simulink model "lab"  (R2024a)
settings: Solver=ode4  StartTime=0.0  StopTime=50  FixedStep=0.001  RelTol=1e-3
undefined symbols (not defined in the file or in its folder): sigbuilder_block
libraries: slpidlib x1
settings Model: Creator=colom  LastModifiedBy=guilherme
settings SolverCC: AlgebraicLoopSolver=TrustRegion  AutoInsertRateTranBlk=on
settings OptimizationCC: LifeSpan=inf
settings DebuggingCC: SFExecutionAtInitializationDiag=none  ArithmeticOperatorsInVariantConditions=warning
settings HardwareCC: ProdBitPerSizeT=32  ProdBitPerPtrDiffT=32  ProdWordSize=32  ProdHWDeviceType=Specified
settings SFSimCC: CustomCodeUndefinedFunction=UseInterfaceOnly
settings RTWCC: GPUComputeCapability=3.5
settings CodeAppCC: StateflowObjectComments=on

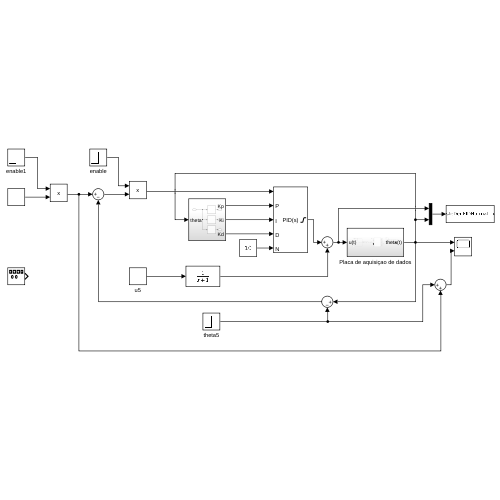
[thumbnail: Simulink's stored preview of the top-level diagram]
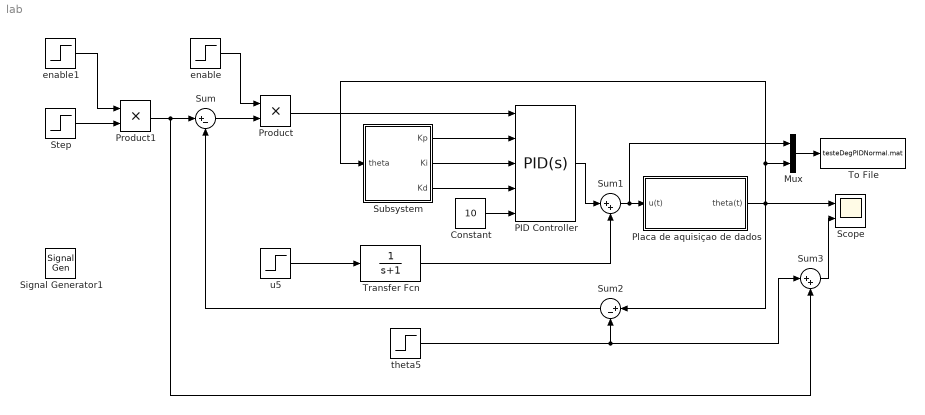
== system lab ==
  Constant : Constant  Value=10
  Mux : Mux  Inputs=2
  PID Controller : slpidlib/PID Controller  Controller=PID  Form=Parallel  TimeDomain=Continuous-time  UseExternalTs=off  SampleTime=-1  IntegratorMethod=Forward Euler  FilterMethod=Forward Euler  ControllerParametersSource=external  P=-0.9  I=60  UseKiTs=off  D=2.15  UseExternalDerivativeSource=off  N=10  UseFilter=on  TunerSelectOption=Transfer Function Based (PID Tuner App)  InitialConditionSource=internal  InitialConditionForIntegrator=0  InitialConditionForFilter=0  DifferentiatorICPrevScaledInput=0  ExternalReset=none  TrackingMode=off  Kt=1  LimitOutput=on  SatLimitsSource=internal  UpperSaturationLimit=85  LowerSaturationLimit=-15  LinearizeAsGain=on  AntiWindupMode=back-calculation  Kb=1  LimitIntegrator=off  UpperIntegratorSaturationLimit=inf  LowerIntegratorSaturationLimit=-inf  POutMin=[]  POutMax=[]  IOutMin=[]  IOutMax=[]  DOutMin=[]  DOutMax=[]  NOutMin=[]  NOutMax=[]  SumOutMin=[]  SumOutMax=[]  SaturationOutMin=[]  SaturationOutMax=[]  PParamMin=[]  PParamMax=[]  IParamMin=[]  IParamMax=[]  DParamMin=[]  DParamMax=[]  NParamMin=[]  NParamMax=[]  KbParamMin=[]  KbParamMax=[]  KtParamMin=[]  KtParamMax=[]  KbOutMin=[]  KbOutMax=[]  KtOutMin=[]  KtOutMax=[]  IntegratorOutMin=[]  IntegratorOutMax=[]  FilterOutMin=[]  FilterOutMax=[]  SumI1OutMin=[]  SumI1OutMax=[]  SumI2OutMin=[]  SumI2OutMax=[]  SumI3OutMin=[]  SumI3OutMax=[]  SumI4OutMin=[]  SumI4OutMax=[]  SumDOutMin=[]  SumDOutMax=[]  DifferentiatorOutMin=[]  DifferentiatorOutMax=[]  FilterDiffOutCoefMin=[]  FilterDiffOutCoefMax=[]  ReciprocalOutMin=[]  ReciprocalOutMax=[]  SumDenOutMin=[]  SumDenOutMax=[]  SumNumOutMin=[]  SumNumOutMax=[]  DivideOutMin=[]  DivideOutMax=[]  UdiffTsProdOutMin=[]  UdiffTsProdOutMax=[]  NTsProdOutMin=[]  NTsProdOutMax=[]  UintegralTsProdOutMin=[]  UintegralTsProdOutMax=[]  UngainTsProdOutMin=[]  UngainTsProdOutMax=[]  ClampingZeroOutDataTypeStr=Inherit: Inherit via back propagation  ClampingZeroOutMin=[]  ClampingZeroOutMax=[]  FilterDenConstantOutDataTypeStr=Inherit: Inherit via back propagation  FilterDenConstantOutMin=[]  FilterDenConstantOutMax=[]  PCopyOutDataTypeStr=Inherit: Inherit via back propagation  PCopyOutMin=[]  PCopyOutMax=[]  NCopyOutDataTypeStr=Inherit: Inherit via back propagation  NCopyOutMin=[]  NCopyOutMax=[]  IntegratorContinuousStateAttributes=''  IntegratorStateMustResolveToSignalObject=off  IntegratorRTWStateStorageClass=Auto  FilterContinuousStateAttributes=''  FilterStateMustResolveToSignalObject=off  FilterRTWStateStorageClass=Auto  ParallelPVariant=ExternalParameters  IdealPVariant=Disabled  IVariant=ExternalParameters  DVariant=ExternalParameters  IntegratorVariant=Continuous  SatVariant=Enabled  AWVariant=BackCalculation  PCopyVariant=Disabled  TRVariant=Disabled  FdbkBlocksVariant=Forward  IdealPFdbkVariant=Disabled  SatFdbkVariant=Disabled  DerivativeFilterVariant=ContFilter  NVariant=ExternalParameters  NCopyVariant=Disabled  FilterICVariant=InternalICsFilter  IntegratorICVariant=InternalICs  ExternalResetVariant=Disabled  TRSumVariant=Passthrough  SumFdbkVariant=Disabled  SumVariant=Sum_PID  TsampFilterVariant=InternalTs  TsampNgainVariant=Passthrough  TsampIntegralVariant=Disabled_SignalSpec  ExternalSaturationOutDataTypeStr=Inherit: Same as second input  DerivativeSourceVariant=ErrorSignal
  Placa de aquisiçao de dados : Subsystem
  Product : Product
  Product1 : Product
  Scope : Scope  NumInputPorts=2
  Signal Generator1 : SignalGenerator  WaveForm=square  Amplitude=deg2rad(10)  Frequency=0.4  Units=rad/sec
  Step : Step  Time=23  After=deg2rad(42)  SampleTime=0
  Subsystem : Subsystem
  Sum : Sum  Inputs=|+-
  Sum1 : Sum  Inputs=|++
  Sum2 : Sum  Inputs=|+-
  Sum3 : Sum  Inputs=|++
  To File : ToFile  Filename=testeDegPIDNormal.mat
      settings: Decimation=3
  Transfer Fcn : TransferFcn  Denominator=[1 1]
  enable : Step  Time=23  SampleTime=0
  enable1 : Step  Time=0  SampleTime=0
  theta5 : Step  Time=16  After=0  SampleTime=0
  u5 : Step  Time=16  After=0  SampleTime=0
  wires:
  Placa de aquisiçao de dados/1(theta(t)) -> Scope/1, Sum2/1, Subsystem/1(theta), Mux/2
  Mux/1 -> To File/1
  u5/1 -> Transfer Fcn/1
  Sum2/1 -> Sum/2
  theta5/1 -> Sum3/1, Sum2/2
  Product/1 -> PID Controller/1
  enable/1 -> Product/1
  Transfer Fcn/1 -> Sum1/2
  Sum1/1 -> Mux/1, Placa de aquisiçao de dados/1(u(t))
  Sum3/1 -> Scope/2
  Sum/1 -> Product/2
  PID Controller/1 -> Sum1/1
  Subsystem/1(Kp) -> PID Controller/2
  Subsystem/2(Ki) -> PID Controller/3
  Subsystem/3(Kd) -> PID Controller/4
  Constant/1 -> PID Controller/5
  Step/1 -> Product1/2
  enable1/1 -> Product1/1
  Product1/1 -> Sum3/2, Sum/1

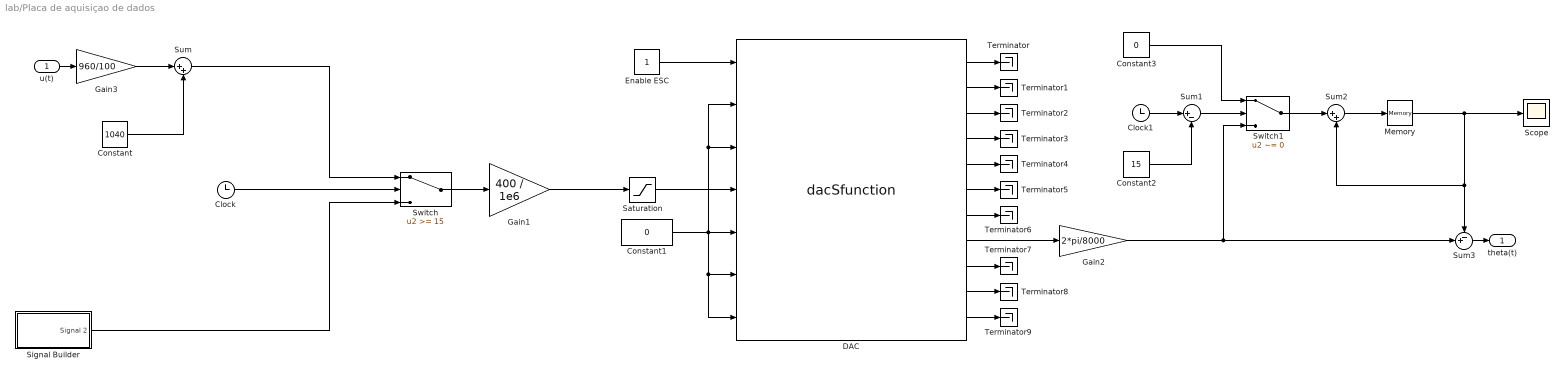
== system lab/Placa de aquisiçao de dados ==
  u(t) : Inport
  Clock : Clock
  Clock1 : Clock
  Constant : Constant  Value=1040
  Constant1 : Constant  Value=0
  Constant2 : Constant  Value=15
  Constant3 : Constant  Value=0
  DAC : S-Function  FunctionName=dacSfunction  Parameters=serialPort,sampleTime,gpioOutCh1FinalState,gpioOutCh2FinalState,gpioOutCh3FinalState,pwmFrequency,pwmCh1FinalDuty,pwmCh2FinalDuty,pwmCh3FinalDuty,pwmCh4FinalDuty,enc1Mode,enc1ResetCount,enc1Direction,enc1Quadrature,enc1Filter,enc2Mode,enc2ResetCount,enc2Direction,enc2Quadrature,enc2Filter,enc3Mode,enc3ResetCount,enc3Direction,enc3Quadrature,enc3Filter  SFunctionDeploymentMode=off  EnableBusSupport=off  mask{serialPort='/dev/ttyACM0', sampleTime=5, gpioOutCh1FinalState=Low, gpioOutCh2FinalState=Low, gpioOutCh3FinalState=Low, pwmFrequency=400, pwmCh1FinalDuty=0, pwmCh2FinalDuty=0, pwmCh3FinalDuty=0, pwmCh4FinalDuty=0, enc1Mode=Counter, enc1Direction=Counter Clock Wise is positive, enc1Quadrature=High resolution, enc1Filter=15, enc1ResetCount=on, enc2Mode=Counter, enc2Direction=Counter Clock Wise is positive, enc2Quadrature=High resolution, enc2Filter=15, enc2ResetCount=off, enc3Mode=Counter, enc3Direction=Clock Wise is positive, enc3Quadrature=High resolution, enc3Filter=15, enc3ResetCount=off}
      mask prompts: serialPort "Serial port"; sampleTime "Sample time (ms)"; gpioOutCh1FinalState "Final state"; gpioOutCh2FinalState "Final state"; gpioOutCh3FinalState "Final state"; pwmFrequency "Frequency (Hz)"; pwmCh1FinalDuty "Final duty"; pwmCh2FinalDuty "Final duty"; pwmCh3FinalDuty "Final duty"; pwmCh4FinalDuty "Final duty"; enc1Mode "Mode"; enc1Direction "Direction"; enc1Quadrature "Resolution"; enc1Filter "Filter"; enc1ResetCount "Reset count"; enc2Mode "Mode"; enc2Direction "Direction"; enc2Quadrature "Resolution"; enc2Filter "Filter"; enc2ResetCount "Reset count"; enc3Mode "Mode"; enc3Direction "Direction"; enc3Quadrature "Resolution"; enc3Filter "Filter"; enc3ResetCount "Reset count"
      mask init:
      | % The first list item is initiated with 1 and not 0
      mask TypeOptions gpioOutCh1FinalState: Low | High
      mask TypeOptions gpioOutCh2FinalState: Low | High
      mask TypeOptions gpioOutCh3FinalState: Low | High
      mask TypeOptions enc1Mode: Counter | Time measurement
      mask TypeOptions enc1Direction: Counter Clock Wise is positive | Clock Wise is positive
      mask TypeOptions enc1Quadrature: Low resolution | High resolution
      mask TypeOptions enc2Mode: Counter | Time measurement
      mask TypeOptions enc2Direction: Counter Clock Wise is positive | Clock Wise is positive
      mask TypeOptions enc2Quadrature: Low resolution | High resolution
      mask TypeOptions enc3Mode: Counter | Time measurement
      mask TypeOptions enc3Direction: Counter Clock Wise is positive | Clock Wise is positive
      mask TypeOptions enc3Quadrature: Low resolution | High resolution
      mask DialogControl DescTextVar Prompt: %<MaskDescription> OpenDAC configuration
      mask DialogControl Container18 Prompt: General configuration
      mask DialogControl Container8 Prompt: GPIO Output
      mask DialogControl Container19 Prompt: Channel 1
      mask DialogControl Container22 Prompt: Channel 2
      mask DialogControl Container21 Prompt: Channel 3
      mask DialogControl Container6 Prompt: PWM
      mask DialogControl Container42 Prompt: General
      mask DialogControl Container43 Prompt: Channel 1
      mask DialogControl pwmCh1FinalDuty Tooltip: 0 - 100%
      mask DialogControl Container11 Prompt: Channel 2
      mask DialogControl pwmCh2FinalDuty Tooltip: 0 - 100%
      mask DialogControl Container12 Prompt: Channel 3
      mask DialogControl pwmCh3FinalDuty Tooltip: 0 - 100%
      mask DialogControl Container13 Prompt: Channel 4
      mask DialogControl pwmCh4FinalDuty Tooltip: 0 - 100%
      mask DialogControl Container4 Prompt: Encoders
      mask DialogControl Container35 Prompt: Encoder 1
      mask DialogControl enc1Quadrature Tooltip: In pulse count mode, Low resolution implements X2 quadrature and High resolution implements X4 quadrature. In time measurement mode, Low Resolution measure time between two rise edges on CHA and High Resolution measure time between rise and fall edges on CHA.
      mask DialogControl Container36_copy Prompt: Encoder 2
      mask DialogControl enc2Quadrature Tooltip: In pulse count mode, Low resolution implements X2 quadrature and High resolution implements X4 quadrature. In time measurement mode, Low Resolution measure time between two rise edges on CHA and High Resolution measure time between rise and fall edges on CHA.
      mask DialogControl Container36 Prompt: Encoder 3
      mask DialogControl enc3Quadrature Tooltip: In pulse count mode, Low resolution implements X2 quadrature and High resolution implements X4 quadrature. In time measurement mode, Low Resolution measure time between two rise edges on CHA and High Resolution measure time between rise and fall edges on CHA.
      mask Display:
      | % Give names to the input ports
      | port_label('input', 1, 'Digital Out CH1 (PC15)');
      | port_label('input', 2, 'Digital Out CH2 (PC14)');
      | port_label('input', 3, 'Digital Out CH3 (PC13)');
      | port_label('input', 4, 'PWM CH1 (PB6)');
      | port_label('input', 5, 'PWM CH2 (PB7)');
      | port_label('input', 6, 'PWM CH3 (PB8)');
      | port_label('input', 7, 'PWM CH4 (PB9)');
      | 
      | % Give names to the output ports
      | port_label('output', 1, 'Digital In CH1 (PB12)');
      | port_label('output', 2, 'Digital In CH2 (PB13)');
      | port_label('output', 3, 'Digital In CH3 (PB14)');
      | port_label('output', 4, 'Analog In CH1 (PA0)');
      | port_label('output', 5, 'Analog In CH2 (PA1)');
      | port_label('output', 6, 'Analog In CH3 (PA4)');
      | port_label('output', 7, 'Analog In CH4 (PB0)');
      | port_label('output', 8, 'Encoder 1 (PA8/PA9)');
      | port_label('output', 9, 'Encoder 2 (PA15/PB3)');
      | port_label('output', 10, 'Encoder 3 (PB4/PB5)');
      | port_label('output', 11, 'Real Time Clock');
  Enable ESC : Constant
  Gain1 : Gain  Gain=400 / 1e6
  Gain2 : Gain  Gain=2*pi/8000
  Gain3 : Gain  Gain=960/100
  Memory : Memory
  Saturation : Saturate  UpperLimit=0.8  LowerLimit=0
  Scope : Scope
  Signal Builder : Subsystem  Tag=STV Subsys  LoadFcn=sigbuilder_block('load');  StartFcn=sigbuilder_block('start');  StopFcn=sigbuilder_block('stop');  ClipboardFcn=sigbuilder_block('clipboard');  mask(Sigbuilder block){tuvar=[0:10]}
      mask help: Simulink:masks:SigbuilderBlock_MD
      mask init:
      | if ~strcmp(get_param(bdroot(gcbh),'SimulationStatus'),'stopped') tuvar = sigbuilder_block('maskInit'); end
      settings: CopyFcn=sigbuilder_block('copy');  DeleteFcn=sigbuilder_block('delete');  ModelCloseFcn=sigbuilder_block('modelClose');  PreSaveFcn=sigbuilder_block('preSave');  PauseFcn=sigbuilder_block('pause');  ContinueFcn=sigbuilder_block('continue');  NameChangeFcn=sigbuilder_block('namechange');  OpenFcn=sigbuilder_block('open',[0 33 1440 687.75 ]);  CloseFcn=sigbuilder_block('close');
      mask Display: plot(0, 0, 100, 100,[2, 2, 32, 32, 2], [68, 8, 8, 68, 68],[32, 2], [38, 38], [32, 19, 2],[53, 60, 44], [32, 17, 17, 2],[16, 16, 31, 31]);txt = getActiveGroup(gcbh);text(2, 100, txt,'verticalAlignment', 'top');
  Sum : Sum  Inputs=|++
  Sum1 : Sum  Inputs=|+-
  Sum2 : Sum  Inputs=|++
  Sum3 : Sum  Inputs=-+|
  Switch : Switch  Threshold=15  SaturateOnIntegerOverflow=off  InputSameDT=off
  Switch1 : Switch  Criteria=u2 ~= 0  SaturateOnIntegerOverflow=off  InputSameDT=off
  Terminator{,1..9} (10 alike) : Terminator
  theta(t) : Outport
  wires:
  Saturation/1 -> DAC/4
  Sum1/1 -> Switch1/2
  DAC/7 -> Terminator6/1
  DAC/11 -> Terminator9/1
  DAC/3 -> Terminator2/1
  Switch/1 -> Gain1/1
  Gain3/1 -> Sum/1
  Memory/1 -> Scope/1, Sum2/2, Sum3/1
  Constant1/1 -> DAC/3, DAC/2, DAC/7, DAC/6, DAC/5
  Gain2/1 -> Sum3/2, Switch1/3
  Clock1/1 -> Sum1/1
  DAC/8 -> Gain2/1
  Sum/1 -> Switch/1
  DAC/2 -> Terminator1/1
  DAC/9 -> Terminator7/1
  Sum3/1 -> theta(t)/1
  Constant3/1 -> Switch1/1
  DAC/5 -> Terminator4/1
  Constant2/1 -> Sum1/2
  DAC/10 -> Terminator8/1
  Sum2/1 -> Memory/1
  DAC/6 -> Terminator5/1
  DAC/1 -> Terminator/1
  DAC/4 -> Terminator3/1
  Enable ESC/1 -> DAC/1
  u(t)/1 -> Gain3/1
  Switch1/1 -> Sum2/1
  Clock/1 -> Switch/2
  Constant/1 -> Sum/2
  Gain1/1 -> Saturation/1
  Signal Builder/1(Signal 2) -> Switch/3

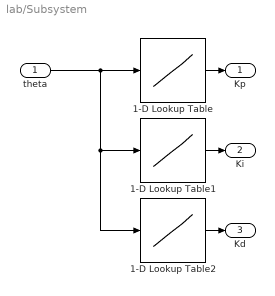
== system lab/Subsystem ==
  theta : Inport
  1-D Lookup Table : Lookup_n-D  NumberOfTableDimensions=1  BreakpointsForDimension1=[0.114;0.3862;0.6568;0.9247]  Table=[-3.4242;-4.0295;-2.3476;2.6465]  InternalRulePriority=Speed  RndMeth=Simplest
  1-D Lookup Table1 : Lookup_n-D  NumberOfTableDimensions=1  BreakpointsForDimension1=[0.114;0.3862;0.6568;0.9247]  Table=[46.3166;62.1752;69.7699;81.9909]  InternalRulePriority=Speed  RndMeth=Simplest
  1-D Lookup Table2 : Lookup_n-D  NumberOfTableDimensions=1  BreakpointsForDimension1=[0.114;0.3862;0.6568;0.9247]  Table=[1.6110;2.4421;3.2407;4.9246]  InternalRulePriority=Speed  RndMeth=Simplest
  Kp : Outport
  Ki : Outport  Port=2
  Kd : Outport  Port=3
  wires:
  1-D Lookup Table1/1 -> Ki/1
  1-D Lookup Table2/1 -> Kd/1
  1-D Lookup Table/1 -> Kp/1
  theta/1 -> 1-D Lookup Table2/1, 1-D Lookup Table1/1, 1-D Lookup Table/1

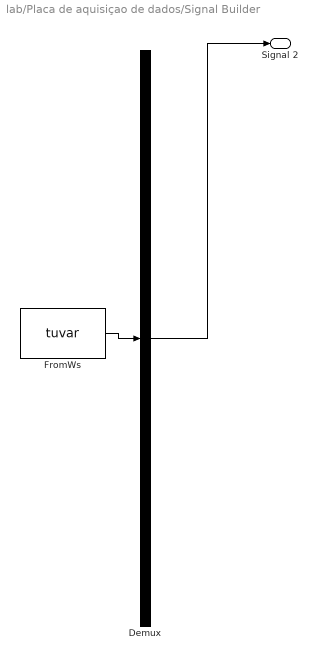
== system lab/Placa de aquisiçao de dados/Signal Builder ==
  Demux : Demux  Tag=STV Demux  Outputs=1
      settings: DisplayOption=none
  FromWs : FromWorkspace  Tag=STV FromWs  VariableName=tuvar
      SigBuilderData=|
      | common.afterFinalStr = 'Extrapolate'
      | common.sampleTime = 0
      | dataSet.timeRange = [0 20]
      | dataSet.name = 'Group 1'
      | sbobj.Groups.Name = 'Group 1'
      | sbobj.Groups.Signals.Name = 'Signal 2'
      | sbobj.Groups.Signals.XData = [0 1 1 3 3 7 7 20]
      | sbobj.Groups.Signals.YData = [0 0 2000 2000 0 0 1040 1040]
      | sbobj.Groups.TimeRange = [0 20]
  Signal 2 : Outport  Tag=STV Outport
  wires:
  FromWs/1 -> Demux/1
  Demux/1 -> Signal 2/1
